simulink model "sim_mcce_scheduled_control"  (R2016a)
settings: Solver=VariableStepAuto  StartTime=0.0  StopTime=1  RelTol=1e-5
values from neighbouring files (symbols this model uses):
  Ts = 4e-4    (= 0.0004)    [calculate_gains.m]    (also in generate_lookup_table.m = 0.0005)
  ws_lt = -30000 : 2500 :30000    [generate_lookup_table.m]
undefined symbols (not defined in the file or in its folder): Ad_lt, Bd_lt, Cd_lt, DiscIntNeverNeededParam, Kdi_lt, Kdo_lt
settings Model: Creator=manuel  LastModifiedBy=manuel

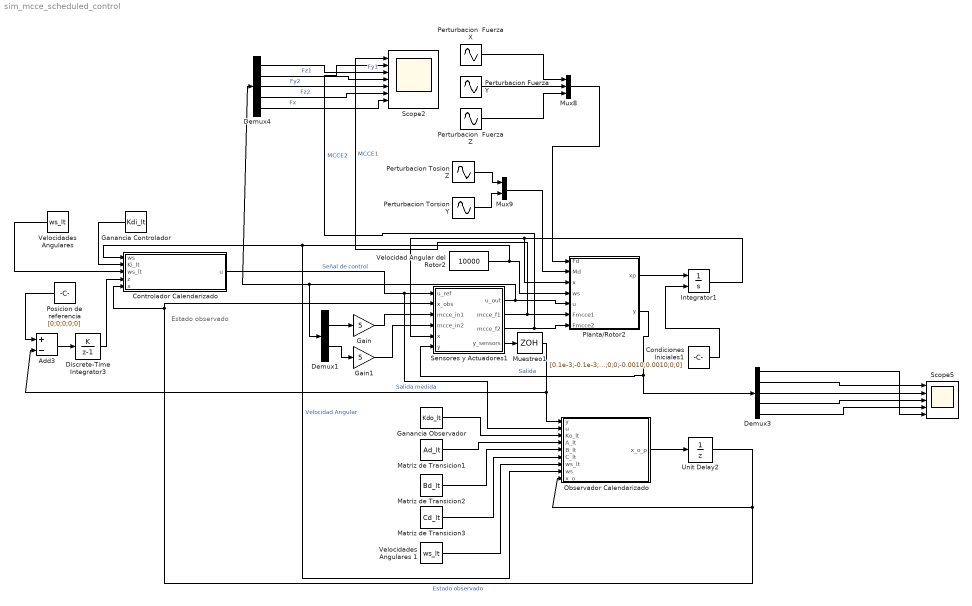
== system sim_mcce_scheduled_control ==
  note: Estado observado
  Add3 : Sum  Inputs=+-
  Condiciones Iniciales1 : Constant  Value=[0.1e-3;-0.1e-3;0.1e-3;0;0;0;-0.0010;0.0010;0;0]
  Controlador Calendarizado : MATLAB Function  TreatAsAtomicUnit=on
  Demux1 : Demux  Outputs=5
  Demux3 : Demux  Outputs=5
  Demux4 : Demux  Outputs=5
  Discrete-Time Integrator3 : DiscreteIntegrator  IntegratorMethod=Accumulation: Forward Euler  gainval=1  InitialCondition=[0;0;0;0;0]  InitialConditionSetting=State (most efficient)  SampleTime=-1  ICPrevOutput=DiscIntNeverNeededParam  ICPrevScaledInput=DiscIntNeverNeededParam
  Gain : Gain  Gain=5
  Gain1 : Gain  Gain=5
  Ganancia Controlador : Constant  Value=Kdi_lt  VectorParams1D=off
  Ganancia Observador : Constant  Value=Kdo_lt  VectorParams1D=off
  Integrator1 : Integrator  InitialConditionSource=external  InitialCondition=[0;0;0;0;0;0;0;0;0;0]
  Matriz de Transicion1 : Constant  Value=Ad_lt  VectorParams1D=off
  Matriz de Transicion2 : Constant  Value=Bd_lt  VectorParams1D=off
  Matriz de Transicion3 : Constant  Value=Cd_lt  VectorParams1D=off
  Muestreo1 : ZeroOrderHold  SampleTime=Ts
  Mux8 : Mux  Inputs=3
  Mux9 : Mux  Inputs=2
  Observador Calendarizado : MATLAB Function  TreatAsAtomicUnit=on
  Perturbacion  Fuerza X : Sin  Frequency=50*2*pi  SampleTime=0
  Perturbacion  Fuerza Z : Sin  Amplitude=3  Bias=-25  Frequency=100*2*pi  SampleTime=0
  Perturbacion Fuerza Y : Sin  Frequency=100*2*pi  SampleTime=0
  Perturbacion Torsion Y : Sin  Amplitude=0  Frequency=300*2*pi  SampleTime=0
  Perturbacion Tosion Z : Sin  Amplitude=0  Frequency=600*2*pi  SampleTime=0
  Planta/Rotor2 : MATLAB Function  TreatAsAtomicUnit=on
  Posicion de referencia : Constant  Value=[0;0;0;0;0]
  Scope2 : Scope  NumInputPorts=7
  Scope5 : Scope  NumInputPorts=5
  Sensores y Actuadores1 : Subsystem
  Unit Delay2 : UnitDelay  InitialCondition=[0;0;0;0;0;0;0;0;0;0]  SampleTime=-1
  Velocidad Angular del Rotor2 : Constant  Value=10000  VectorParams1D=off
  Velocidades Angulares : Constant  Value=ws_lt  VectorParams1D=off
  Velocidades Angulares 1 : Constant  Value=ws_lt  VectorParams1D=off
  wires:
  Demux4/1 -> Scope2/3  "Fy1"
  Demux4/2 -> Scope2/4  "Fz1"
  Demux4/3 -> Scope2/5  "Fy2"
  Demux4/4 -> Scope2/6  "Fz2"
  Demux4/5 -> Scope2/7  "Fx"
  Ganancia Controlador/1 -> Controlador Calendarizado/2(Ki_lt)
  Ganancia Observador/1 -> Observador Calendarizado/3(Ko_lt)
  Matriz de Transicion1/1 -> Observador Calendarizado/4(A_lt)
  Matriz de Transicion2/1 -> Observador Calendarizado/5(B_lt)
  Matriz de Transicion3/1 -> Observador Calendarizado/6(C_lt)
  Velocidades Angulares/1 -> Controlador Calendarizado/3(ws_lt)
  Velocidades Angulares 1/1 -> Observador Calendarizado/7(ws_lt)
  Integrator1/1 -> Sensores y Actuadores1/5(x), Planta/Rotor2/3(x)
  Planta/Rotor2/1(xp) -> Integrator1/1
  Posicion de referencia/1 -> Add3/1
  Unit Delay2/1 -> Observador Calendarizado/9(x_o), Sensores y Actuadores1/2(x_obs), Controlador Calendarizado/5(x)  "Estado observado"
  Gain/1 -> Sensores y Actuadores1/3(mcce_in1)
  Gain1/1 -> Sensores y Actuadores1/4(mcce_in2)
  Sensores y Actuadores1/3(mcce_f2) -> Planta/Rotor2/7(Fmcce2), Scope2/2  "MCCE2"
  Planta/Rotor2/2(y) -> Demux3/1, Sensores y Actuadores1/6(y)  "Salida"
  Sensores y Actuadores1/4(y_sensors) -> Muestreo1/1
  Condiciones Iniciales1/1 -> Integrator1/2
  Muestreo1/1 -> Observador Calendarizado/1(y), Add3/2  "Salida medida"
  Add3/1 -> Discrete-Time Integrator3/1
  Observador Calendarizado/1(x_o_p) -> Unit Delay2/1
  Discrete-Time Integrator3/1 -> Controlador Calendarizado/4(z)
  Velocidad Angular del Rotor2/1 -> Controlador Calendarizado/1(ws), Observador Calendarizado/8(ws), Planta/Rotor2/4(ws)  "Velocidad Angular"
  Demux1/2 -> Gain/1
  Demux1/4 -> Gain1/1
  Controlador Calendarizado/1(u) -> Observador Calendarizado/2(u), Sensores y Actuadores1/1(u_ref)  "Señal de control"
  Mux9/1 -> Planta/Rotor2/2(Md)
  Mux8/1 -> Planta/Rotor2/1(Fd)
  Perturbacion Tosion Z/1 -> Mux9/1
  Perturbacion Torsion Y/1 -> Mux9/2
  Perturbacion Fuerza Y/1 -> Mux8/2
  Perturbacion  Fuerza Z/1 -> Mux8/3
  Perturbacion  Fuerza X/1 -> Mux8/1
  Demux3/1 -> Scope5/5
  Demux3/2 -> Scope5/1
  Demux3/3 -> Scope5/2
  Demux3/4 -> Scope5/3
  Demux3/5 -> Scope5/4
  Sensores y Actuadores1/1(u_out) -> Demux1/1, Demux4/1, Planta/Rotor2/5(u)
  Sensores y Actuadores1/2(mcce_f1) -> Scope2/1, Planta/Rotor2/6(Fmcce1)  "MCCE1"

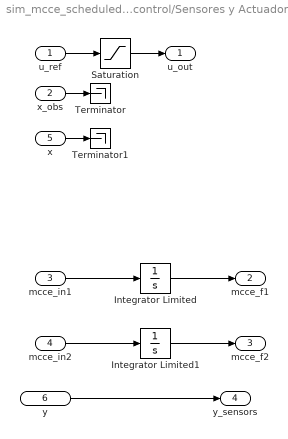
== system sim_mcce_scheduled_control/Sensores y Actuadores1 ==
  u_ref : Inport
  x_obs : Inport  Port=2
  mcce_in1 : Inport  Port=3
  mcce_in2 : Inport  Port=4
  x : Inport  Port=5
  y : Inport  Port=6
  Integrator Limited : Integrator  InitialCondition=6  LimitOutput=on  UpperSaturationLimit=40  LowerSaturationLimit=6
  Integrator Limited1 : Integrator  InitialCondition=6  LimitOutput=on  UpperSaturationLimit=40  LowerSaturationLimit=6
  Saturation : Saturate  UpperLimit=50  LowerLimit=-50
  Terminator : Terminator
  Terminator1 : Terminator
  u_out : Outport
  mcce_f1 : Outport  Port=2
  mcce_f2 : Outport  Port=3
  y_sensors : Outport  Port=4
  wires:
  y/1 -> y_sensors/1
  x/1 -> Terminator1/1
  Integrator Limited1/1 -> mcce_f2/1
  mcce_in2/1 -> Integrator Limited1/1
  mcce_in1/1 -> Integrator Limited/1
  Integrator Limited/1 -> mcce_f1/1
  x_obs/1 -> Terminator/1
  u_ref/1 -> Saturation/1
  Saturation/1 -> u_out/1

== matlab function sim_mcce_scheduled_control/Observador Calendarizado ==
  data: y input; u input; x_o_p output; Ko_lt input; A_lt input; B_lt input; C_lt input; ws_lt input; ws input; x_o input
function x_o_p = state_obsever(y,u,Ko_lt,A_lt,B_lt,C_lt,ws_lt,ws,x_o)
%#codegen
Ko = matrix_interpolation(ws_lt,Ko_lt,ws);
A = matrix_interpolation(ws_lt,A_lt,ws);
B = matrix_interpolation(ws_lt,B_lt,ws);
C = matrix_interpolation(ws_lt,C_lt,ws);

x_o_p = A*x_o + B*u + Ko*(y-C*x_o);

== matlab function sim_mcce_scheduled_control/Planta//Rotor2 ==
  data: Fd input; Md input; xp output; x input; ws input; y output; u input; Fmcce1 input; Fmcce2 input
function [xp,y]  = fcn(Fd,Md,x,ws,u,Fmcce1,Fmcce2)
Fd_x = Fd(1);
Fd_y = Fd(2);
Fd_z = Fd(3);
Md_y = Md(1);
Md_z = Md(2);
[xp,y] = hmb_non_linear_model(x,u,ws,Fd_x,Fd_y,Fd_z,Md_y,Md_z,Fmcce1,Fmcce2);
end

== matlab function sim_mcce_scheduled_control/Controlador Calendarizado ==
  data: ws input; Ki_lt input; ws_lt input; z input; x input; u output
function u  = feedback_controller(ws,Ki_lt,ws_lt,z,x)
%#codegen
ki = matrix_interpolation(ws_lt,Ki_lt,ws);

xi = [x;z];

u = -ki*xi;
